simulink model "TurnLightArb_backup"  (R2023a)
settings: Solver=FixedStepDiscrete  StartTime=0.0  StopTime=10.0  FixedStep=0.01  RelTol=1e-3
settings Model: Creator=19856  LastModifiedBy=19856
settings DataIOCC: SaveFormat=StructureWithTime
settings OptimizationCC: DefaultParameterBehavior=Inlined  EnhancedBackFolding=on  PassReuseOutputArgsAs=Individual arguments  ZeroExternalMemoryAtStartup=off  ZeroInternalMemoryAtStartup=off  OptimizeBlockOrder=speed  DifferentSizesBufferReuse=on  OptimizationCustomize=off  EfficientTunableParamExpr=on
settings DebuggingCC: ParameterTunabilityLossMsg=error
settings ModelReferenceCC: ModelReferenceNumInstancesAllowed=Single
settings SFSimCC: MATLABDynamicMemAlloc=off
settings RTWCC: Description=AUTOSAR  SystemTargetFile=autosar.tlc  GenCodeOnly=on  TemplateMakefile=ert_default_tmf
settings CodeAppCC: ForceParamTrailComments=on  IgnoreCustomStorageClasses=off  OperatorAnnotations=on  SimulinkDataObjDesc=on  SFDataObjDesc=on  InsertBlockDesc=on
settings STFCustomTargetCC: MultiwordLength=256  ParMdlRefBuildCompliant=on  CompOptLevelCompliant=on  ConcurrentExecutionCompliant=off  IncludeMdlTerminateFcn=off  CombineOutputUpdateFcns=on  SuppressErrorStatus=on  ERTCustomFileBanners=on  SupportNonFinite=off  SupportComplex=off  SupportContinuousTime=off  SupportNonInlinedSFcns=off  RemoveResetFunc=on  MATLABClassNameForMDSCustomization=Simulink.SoftwareTarget.ERTCustomization  AutosarCompliant=on  GRTInterface=off  LookupTableObjectStructAxisOrder=2,1,3,4,...  LUTObjectStructOrderEvenSpacing=Size,Table,Breakpoints  SystemTargetFile=autosar.tlc
settings ERTTargetCC: TargetLangStandard=C99 (ISO)  ConcurrentExecutionCompliant=off  IncludeMdlTerminateFcn=off  SuppressErrorStatus=on  SupportNonFinite=off  SupportComplex=off  ModelStepFunctionPrototypeControlCompliant=off  CPPClassGenCompliant=off  AutosarCompliant=on  LookupTableObjectStructAxisOrder=2,1,3,4,...  LUTObjectStructOrderEvenSpacing=Size,Table,Breakpoints  InlinedParameterPlacement=NonHierarchical  ERTCustomFileTemplate=example_file_process.tlc

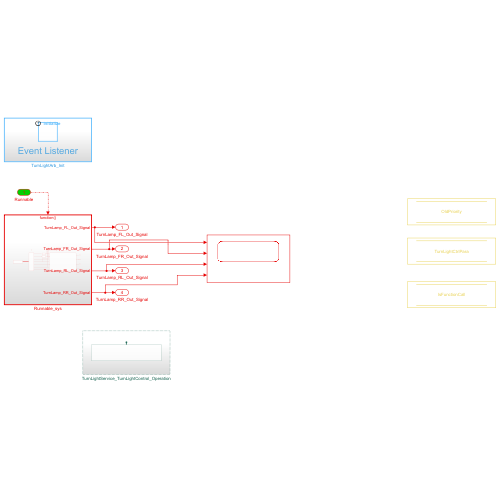
[thumbnail: Simulink's stored preview of the top-level diagram]
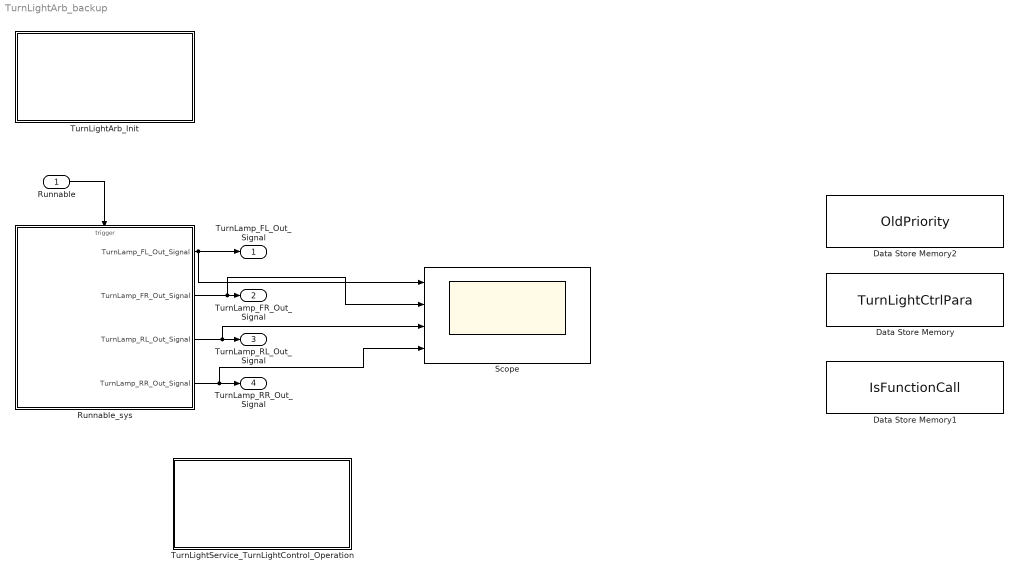
== system TurnLightArb_backup ==
  Runnable : Inport  SampleTime=0.01  OutputFunctionCall=on
  Data Store Memory : DataStoreMemory  DataStoreName=TurnLightCtrlPara  WriteAfterWriteMsg=warning  ShowAdditionalParam=off  OutDataTypeStr=Bus: TurnLightService
  Data Store Memory1 : DataStoreMemory  DataStoreName=IsFunctionCall  WriteAfterWriteMsg=warning  ShowAdditionalParam=off  OutDataTypeStr=boolean
  Data Store Memory2 : DataStoreMemory  DataStoreName=OldPriority  WriteAfterWriteMsg=warning  ShowAdditionalParam=off  OutDataTypeStr=uint8
  Runnable_sys : Subsystem
  Scope : Scope  NumInputPorts=4
  TurnLightArb_Init : Subsystem
  TurnLightService_TurnLightControl_Operation : Subsystem
  TurnLamp_FL_Out_Signal : Outport  OutDataTypeStr=uint8  PortDimensions=1
  TurnLamp_FR_Out_Signal : Outport  Port=2  OutDataTypeStr=uint8  PortDimensions=1
  TurnLamp_RL_Out_Signal : Outport  Port=3  OutDataTypeStr=uint8  PortDimensions=1
  TurnLamp_RR_Out_Signal : Outport  Port=4  OutDataTypeStr=uint8  PortDimensions=1
  wires:
  Runnable_sys/1(TurnLamp_FL_Out_Signal) -> TurnLamp_FL_Out_Signal/1, Scope/1
  Runnable_sys/2(TurnLamp_FR_Out_Signal) -> Scope/2, TurnLamp_FR_Out_Signal/1
  Runnable_sys/3(TurnLamp_RL_Out_Signal) -> Scope/3, TurnLamp_RL_Out_Signal/1
  Runnable/1 -> Runnable_sys/Trigger
  Runnable_sys/4(TurnLamp_RR_Out_Signal) -> Scope/4, TurnLamp_RR_Out_Signal/1

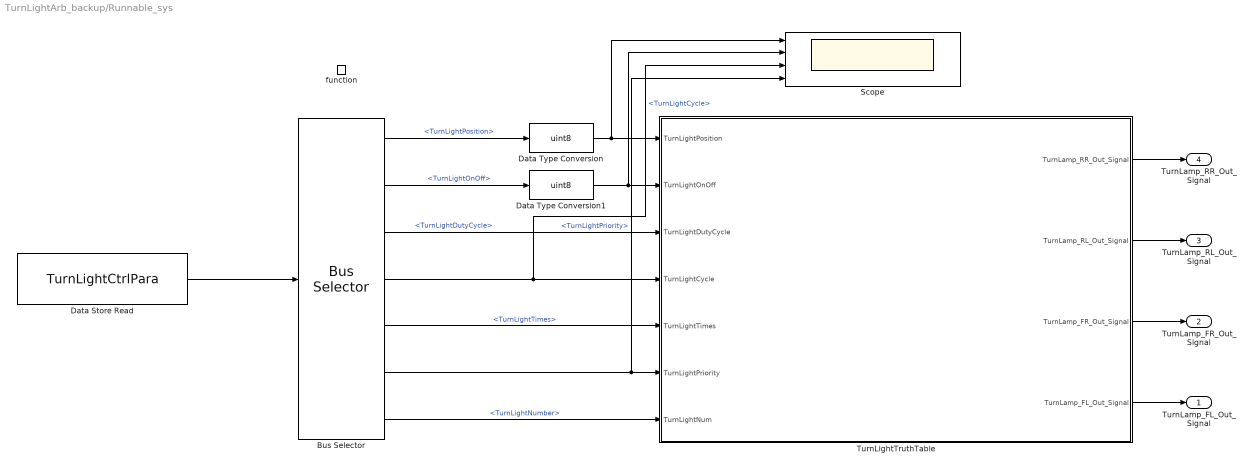
== system TurnLightArb_backup/Runnable_sys ==
  function : TriggerPort  TriggerType=function-call  VariantControl=(inherit)  SampleTimeType=periodic  SampleTime=-1
  Bus Selector : BusSelector  OutputSignals=TurnLightPosition,TurnLightOnOff,TurnLightDutyCycle,TurnLightCycle,TurnLightTimes,TurnLightPriority,TurnLightNumber
  Data Store Read : DataStoreRead  DataStoreName=TurnLightCtrlPara  IndexOptions=Index vector (dialog)  Indices=1  OutputSizes=1
  Data Type Conversion : DataTypeConversion  OutDataTypeStr=uint8  SaturateOnIntegerOverflow=off  RndMeth=Floor
  Data Type Conversion1 : DataTypeConversion  OutDataTypeStr=uint8  SaturateOnIntegerOverflow=off  RndMeth=Floor
  Scope : Scope  NumInputPorts=4
  TurnLightTruthTable : Stateflow chart  TreatAsAtomicUnit=on
      settings: PortSchema="{\"entries\":[{\"content\":{\"sides\":[{\"content\":{\"connectorIds\":[\"In5\",\"In4\",\"In2\",\"In1\",\"In7\",\"In6\",\"In3\"]},\"type\":\"ConnectorPlacement.EquallySpacedRectSide\",\"uuid\":\"5a788a4c-5a8d-43bd-a6c6-e3463c95aa25\"},{\"content\":{\"connectorIds\":[\"Out1\",\"Out2\",\"Out3\",\"Out4\"],\"side\":\"RIGHT\"},\"type\":\"ConnectorPlacement.EquallySpacedRectSide\",\"uuid\":\"f8a0128c-bcbc-49c2-bc1e-8bd751dcd968\"},{\"content\":{\"side\":\"TOP\"},\"type\":\"ConnectorPlacement.EquallySpacedRectSide\",\"uuid\":\"97b9e3af-7316-448b-8a79-903411eabff9\"}]},\"type\":\"ConnectorPlacement.EquallySpacedConnector\",\"uuid\":\"9f734a98-c34a-435a-8c8c-44914ce2cc45\"}],\"packageUris\":[\"http://schema.mathworks.com/mf0/Connector/R2020b\"],\"version\":\"1.0\"}"
  TurnLamp_FL_Out_Signal : Outport
      settings: EnsureOutportIsVirtual=on
  TurnLamp_FR_Out_Signal : Outport  Port=2
      settings: EnsureOutportIsVirtual=on
  TurnLamp_RL_Out_Signal : Outport  Port=3
      settings: EnsureOutportIsVirtual=on
  TurnLamp_RR_Out_Signal : Outport  Port=4
      settings: EnsureOutportIsVirtual=on
  wires:
  TurnLightTruthTable/4(TurnLamp_FL_Out_Signal) -> TurnLamp_FL_Out_Signal/1
  TurnLightTruthTable/3(TurnLamp_FR_Out_Signal) -> TurnLamp_FR_Out_Signal/1
  TurnLightTruthTable/2(TurnLamp_RL_Out_Signal) -> TurnLamp_RL_Out_Signal/1
  TurnLightTruthTable/1(TurnLamp_RR_Out_Signal) -> TurnLamp_RR_Out_Signal/1
  Data Store Read/1 -> Bus Selector/1
  Bus Selector/1 -> Data Type Conversion/1  "<TurnLightPosition>"
  Bus Selector/2 -> Data Type Conversion1/1  "<TurnLightOnOff>"
  Bus Selector/3 -> TurnLightTruthTable/2(TurnLightDutyCycle)  "<TurnLightDutyCycle>"
  Bus Selector/4 -> Scope/3, TurnLightTruthTable/1(TurnLightCycle)  "<TurnLightCycle>"
  Bus Selector/5 -> TurnLightTruthTable/7(TurnLightTimes)  "<TurnLightTimes>"
  Bus Selector/6 -> TurnLightTruthTable/6(TurnLightPriority), Scope/4  "<TurnLightPriority>"
  Data Type Conversion/1 -> Scope/1, TurnLightTruthTable/5(TurnLightPosition)
  Data Type Conversion1/1 -> Scope/2, TurnLightTruthTable/4(TurnLightOnOff)
  Bus Selector/7 -> TurnLightTruthTable/3(TurnLightNum)  "<TurnLightNumber>"

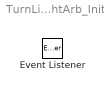
== system TurnLightArb_backup/TurnLightArb_Init ==
  Event Listener : EventListener  EventName=reset

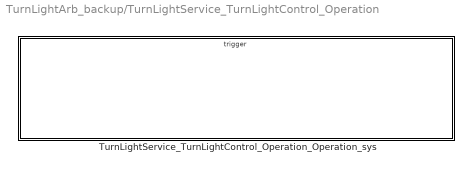
== system TurnLightArb_backup/TurnLightService_TurnLightControl_Operation ==
  TurnLightService_TurnLightControl_Operation_Operation_sys : Subsystem

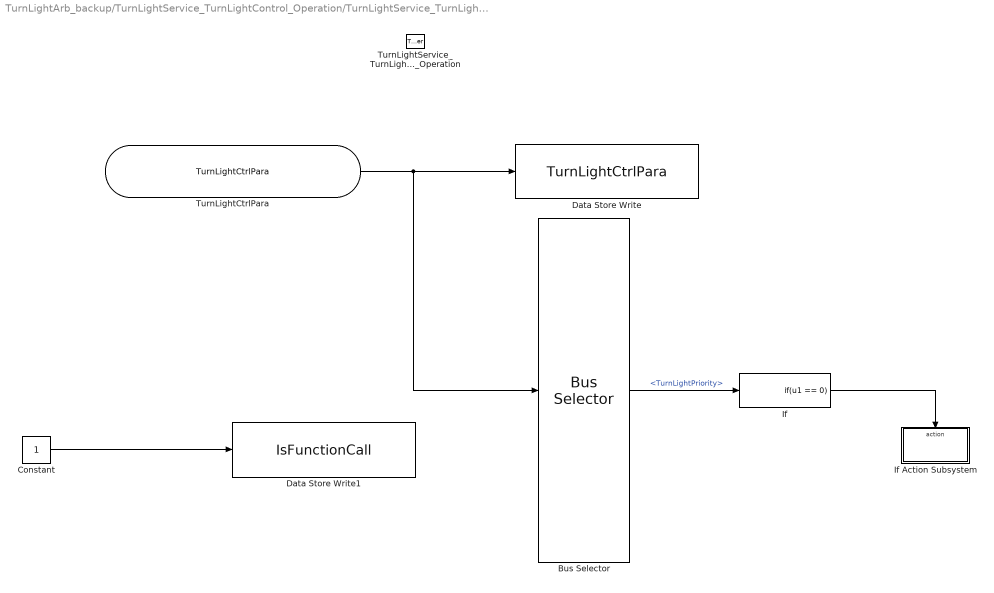
== system TurnLightArb_backup/TurnLightService_TurnLightControl_Operation/TurnLightService_TurnLightControl_Operation_Operation_sys ==
  TurnLightService_TurnLightControl_Operation_Operation : TriggerPort  TriggerType=function-call  IsSimulinkFunction=on  FunctionName=TurnLightService_TurnLightControl_Operation_Operation  VariantControl=(inherit)
  Bus Selector : BusSelector  OutputSignals=TurnLightPriority
  Constant : Constant  OutDataTypeStr=boolean
  Data Store Write : DataStoreWrite  DataStoreName=TurnLightCtrlPara  IndexOptions=Index vector (dialog)  Indices=1  OutputSizes=1
  Data Store Write1 : DataStoreWrite  DataStoreName=IsFunctionCall  IndexOptions=Index vector (dialog)  Indices=1  OutputSizes=1
  If : If  IfExpression=u1 == 0  ShowElse=off
  If Action Subsystem : Subsystem  TreatAsAtomicUnit=on
  TurnLightCtrlPara : ArgIn  OutDataTypeStr=Bus: TurnLightService  ArgumentName=TurnLightCtrlPara
  wires:
  TurnLightCtrlPara/1 -> Bus Selector/1, Data Store Write/1
  Constant/1 -> Data Store Write1/1
  Bus Selector/1 -> If/1  "<TurnLightPriority>"
  If/1 -> If Action Subsystem/Action

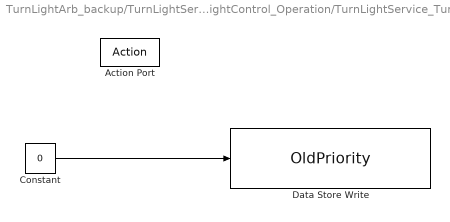
== system TurnLightArb_backup/TurnLightService_TurnLightControl_Operation/TurnLightService_TurnLightControl_Operation_Operation_sys/If Action Subsystem ==
  Action Port : ActionPort  ActionPortLabel=if(u1 == 0)
  Constant : Constant  Value=0  OutDataTypeStr=uint8
  Data Store Write : DataStoreWrite  DataStoreName=OldPriority  IndexOptions=Index vector (dialog)  Indices=1  OutputSizes=1
  wires:
  Constant/1 -> Data Store Write/1

== stateflow chart TurnLightArb_backup/Runnable_sys/TurnLightTruthTable ==
  state IDLE_
    en:
    UsePriorityArb();
  state TrunLightArtribution [function]
    (default) -> (junction 448)
    (junction 448) -> (junction 450) : { aVarTruthTableCondition_1 = (TurnLightPosition==ComplexTurnLightPosition.RIGHT); }
    (junction 450) -> (junction 452) : { aVarTruthTableCondition_2 = (TurnLightPosition==ComplexTurnLightPosition.LEFT); }
    (junction 452) -> (junction 454) : { aVarTruthTableCondition_3 = (TurnLightPosition==ComplexTurnLightPosition.FRONT_LEFT); }
    (junction 454) -> (junction 456) : { aVarTruthTableCondition_4 = (TurnLightPosition==ComplexTurnLightPosition.FRONT_RIGHT); }
    (junction 456) -> (junction 458) : { aVarTruthTableCondition_5 = (TurnLightPosition==ComplexTurnLightPosition.REAR_LEFT); }
    (junction 458) -> (junction 460) : { aVarTruthTableCondition_6 = (TurnLightPosition==ComplexTurnLightPosition.REAR_RIGHT); }
    (junction 460) -> (junction 462) : { aVarTruthTableCondition_7 = (TurnLightPosition==ComplexTurnLightPosition.ALL); }
    (junction 462) -> (junction 464) : { aVarTruthTableCondition_8 = (TurnLightOnOff==ComplexTurnLightOnOff.ON); }
    (junction 464) -> (junction 466) : { aVarTruthTableCondition_9 = (TurnLightOnOff==ComplexTurnLightOnOff.OFF); }
    (junction 466) -> (junction 468) : { aVarTruthTableCondition_10 = (TurnLightCycle==8); }
    (junction 468) -> (junction 470) : { aVarTruthTableCondition_11 = (TurnLightCycle==4); }
    (junction 470) -> (junction 472) : { aVarTruthTableCondition_12 = (TurnLightPriority==3); }
    (junction 472) -> (junction 474) : { aVarTruthTableCondition_13 = (TurnLightPriority==4); }
    (junction 474) -> (junction 476) : { aVarTruthTableCondition_14 = (TurnLightNum==3); }
    (junction 476) -> (junction 478) : { aVarTruthTableCondition_15 = (TurnLightNum==0); }
    (junction 478) -> (junction 480) [order 1] : [aVarTruthTableCondition_3 && aVarTruthTableCondition_9 && aVarTruthTableCondition_13 && aVarTruthTableCondition_15]
    (junction 480) -> (junction 482) : {
        | /* 'FL_OFF': */
        | TurnLamp_FL_Out_Signal=NOQUEST;
        | }
    (junction 478) -> (junction 484) [order 2]
    (junction 484) -> (junction 486) [order 1] : [aVarTruthTableCondition_4 && aVarTruthTableCondition_9 && aVarTruthTableCondition_13 && aVarTruthTableCondition_15]
    (junction 486) -> (junction 488) : {
        | /* 'FR_OFF': */
        | TurnLamp_FR_Out_Signal=NOQUEST;
        | }
    (junction 484) -> (junction 490) [order 2]
    (junction 490) -> (junction 492) [order 1] : [aVarTruthTableCondition_5 && aVarTruthTableCondition_9 && aVarTruthTableCondition_13 && aVarTruthTableCondition_15]
    (junction 492) -> (junction 494) : {
        | /* 'RL_OFF': */
        | TurnLamp_RL_Out_Signal=NOQUEST;
        | }
    (junction 490) -> (junction 496) [order 2]
    (junction 496) -> (junction 498) [order 1] : [aVarTruthTableCondition_6 && aVarTruthTableCondition_9 && aVarTruthTableCondition_13 && aVarTruthTableCondition_15]
    (junction 498) -> (junction 500) : {
        | /* 'RR_OFF': */
        | TurnLamp_RR_Out_Signal=NOQUEST;
        | }
    (junction 496) -> (junction 502) [order 2]
    (junction 502) -> (junction 504) [order 1] : [aVarTruthTableCondition_3 && aVarTruthTableCondition_8 && aVarTruthTableCondition_11 && aVarTruthTableCondition_13 && aVarTruthTableCondition_15]
    (junction 504) -> (junction 506) : {
        | /* 'FL_DOUBLE': */
        | TurnLamp_FL_Out_Signal=MODE_DOUBLE;
        | }
    (junction 502) -> (junction 508) [order 2]
    (junction 508) -> (junction 510) [order 1] : [aVarTruthTableCondition_4 && aVarTruthTableCondition_8 && aVarTruthTableCondition_11 && aVarTruthTableCondition_13 && aVarTruthTableCondition_15]
    (junction 510) -> (junction 512) : {
        | /* 'FR_DOUBLE': */
        | TurnLamp_FR_Out_Signal=MODE_DOUBLE;
        | }
    (junction 508) -> (junction 514) [order 2]
    (junction 514) -> (junction 516) [order 1] : [aVarTruthTableCondition_5 && aVarTruthTableCondition_8 && aVarTruthTableCondition_11 && aVarTruthTableCondition_13 && aVarTruthTableCondition_15]
    (junction 516) -> (junction 518) : {
        | /* 'RL_DOUBLE': */
        | TurnLamp_RL_Out_Signal=MODE_DOUBLE;
        | }
    (junction 514) -> (junction 520) [order 2]
    (junction 520) -> (junction 522) [order 1] : [aVarTruthTableCondition_6 && aVarTruthTableCondition_8 && aVarTruthTableCondition_11 && aVarTruthTableCondition_13 && aVarTruthTableCondition_15]
    (junction 522) -> (junction 524) : {
        | /* 'RR_DOUBLE': */
        | TurnLamp_RR_Out_Signal=MODE_DOUBLE;
        | }
    (junction 520) -> (junction 526) [order 2]
    (junction 526) -> (junction 528) [order 1] : [aVarTruthTableCondition_1 && aVarTruthTableCondition_8 && aVarTruthTableCondition_10 && aVarTruthTableCondition_12 && aVarTruthTableCondition_14]
    (junction 528) -> (junction 530) : {
        | /* 'TurnLight_RightShort': */
        | TurnLamp_FR_Out_Signal=MODE_THREE;
        | TurnLamp_RL_Out_Signal=NOQUEST;
        | TurnLamp_RR_Out_Signal=MODE_THREE;
        | TurnLamp_FL_Out_Signal=NOQUEST;
        | }
    (junction 526) -> (junction 532) [order 2]
    (junction 532) -> (junction 534) [order 1] : [aVarTruthTableCondition_1 && aVarTruthTableCondition_8 && aVarTruthTableCondition_10 && aVarTruthTableCondition_12 && aVarTruthTableCondition_15]
    (junction 534) -> (junction 536) : {
        | /* 'TurnLight_RightLong': */
        | TurnLamp_FR_Out_Signal=MODE_LONG;
        | TurnLamp_RL_Out_Signal=NOQUEST;
        | TurnLamp_RR_Out_Signal=MODE_LONG;
        | TurnLamp_FL_Out_Signal=NOQUEST;
        | }
    (junction 532) -> (junction 538) [order 2]
    (junction 538) -> (junction 540) [order 1] : [aVarTruthTableCondition_2 && aVarTruthTableCondition_8 && aVarTruthTableCondition_10 && aVarTruthTableCondition_12 && aVarTruthTableCondition_14]
    (junction 540) -> (junction 542) : {
        | /* 'TurnLight_LeftShort': */
        | TurnLamp_FR_Out_Signal=NOQUEST;
        | TurnLamp_RL_Out_Signal=MODE_THREE;
        | TurnLamp_RR_Out_Signal=NOQUEST;
        | TurnLamp_FL_Out_Signal=MODE_THREE;
        | }
    (junction 538) -> (junction 544) [order 2]
    (junction 544) -> (junction 546) [order 1] : [aVarTruthTableCondition_2 && aVarTruthTableCondition_8 && aVarTruthTableCondition_10 && aVarTruthTableCondition_12 && aVarTruthTableCondition_15]
    (junction 546) -> (junction 548) : {
        | /* 'TurnLight_LeftLong': */
        | TurnLamp_FR_Out_Signal=NOQUEST;
        | TurnLamp_RL_Out_Signal=MODE_LONG;
        | TurnLamp_RR_Out_Signal=NOQUEST;
        | TurnLamp_FL_Out_Signal=MODE_LONG;
        | }
    (junction 544) -> (junction 550) [order 2]
    (junction 550) -> (junction 552) [order 1] : [aVarTruthTableCondition_7 && aVarTruthTableCondition_8 && aVarTruthTableCondition_10 && aVarTruthTableCondition_12 && aVarTruthTableCondition_15]
    (junction 552) -> (junction 554) : {
        | /* 'TurnLight_ALLON': */
        | TurnLamp_FR_Out_Signal=MODE_LONG;
        | TurnLamp_RL_Out_Signal=MODE_LONG;
        | TurnLamp_RR_Out_Signal=MODE_LONG;
        | TurnLamp_FL_Out_Signal=MODE_LONG;
        | }
    (junction 550) -> (junction 556) [order 2]
    (junction 556) -> (junction 558) : [aVarTruthTableCondition_7 && aVarTruthTableCondition_9 && aVarTruthTableCondition_12 && aVarTruthTableCondition_15]
    (junction 558) -> (junction 560) : {
        | /* 'TurnLight_ALLOFF': */
        | TurnLamp_FR_Out_Signal=NOQUEST;
        | TurnLamp_RL_Out_Signal=NOQUEST;
        | TurnLamp_RR_Out_Signal=NOQUEST;
        | TurnLamp_FL_Out_Signal=NOQUEST;
        | }
  state UsePriorityArb [function]
    (default) -> (junction 33)
    (junction 33) -> (junction 34) [order 1] : [OldPriority<=TurnLightPriority]
    (junction 33) -> (junction 35) [order 2]
    (junction 34) -> (junction 36) : {TrunLightArtribution();
        | OldPriority=TurnLightPriority;}
    (junction 36) -> (junction 35)
    (junction 35) -> (junction 37) : {IsFunctionCall=0;}
  (default) -> IDLE_
  IDLE_ -> IDLE_ : [IsFunctionCall==1]
  data: aVarTruthTableCondition_1 temporary boolean =0; aVarTruthTableCondition_2 temporary boolean =0; aVarTruthTableCondition_3 temporary boolean =0; aVarTruthTableCondition_4 temporary boolean =0; aVarTruthTableCondition_5 temporary boolean =0; aVarTruthTableCondition_6 temporary boolean =0; aVarTruthTableCondition_7 temporary boolean =0; aVarTruthTableCondition_8 temporary boolean =0; aVarTruthTableCondition_9 temporary boolean =0; aVarTruthTableCondition_10 temporary boolean =0; aVarTruthTableCondition_11 temporary boolean =0; aVarTruthTableCondition_12 temporary boolean =0; aVarTruthTableCondition_13 temporary boolean =0; aVarTruthTableCondition_14 temporary boolean =0; aVarTruthTableCondition_15 temporary boolean =0; TurnLightCycle input uint8; TurnLightDutyCycle input uint8; TurnLightNum input uint8; TurnLightOnOff input uint8; TurnLightPosition input uint8; TurnLightPriority input uint8; TurnLightTimes input uint8; TurnLamp_RR_Out_Signal output uint8; TurnLamp_RL_Out_Signal output uint8; TurnLamp_FR_Out_Signal output uint8; TurnLamp_FL_Out_Signal output uint8; IsFunctionCall data_store_memory; OldPriority data_store_memory; MODE_DOUBLE constant uint8 =3; MODE_LONG constant uint8 =2; MODE_THREE constant uint8 =1; NOQUEST constant uint8 =0
